simulink model "AGMD"  (R2024b)
settings: Solver=VariableStepAuto  StartTime=0.0  StopTime=10.0  RelTol=1e-3
settings Model: Creator=Jan.Seemann  LastModifiedBy=Jan.Seemann

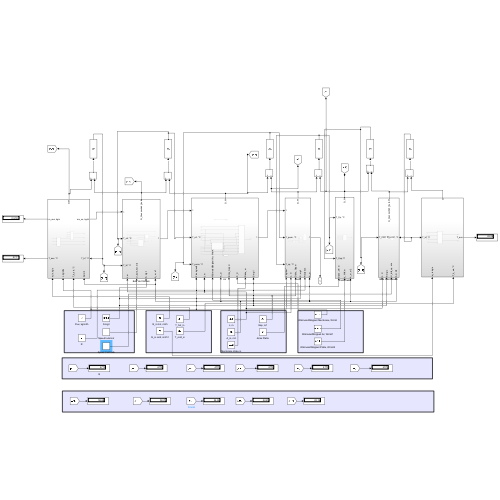
[thumbnail: Simulink's stored preview of the top-level diagram]
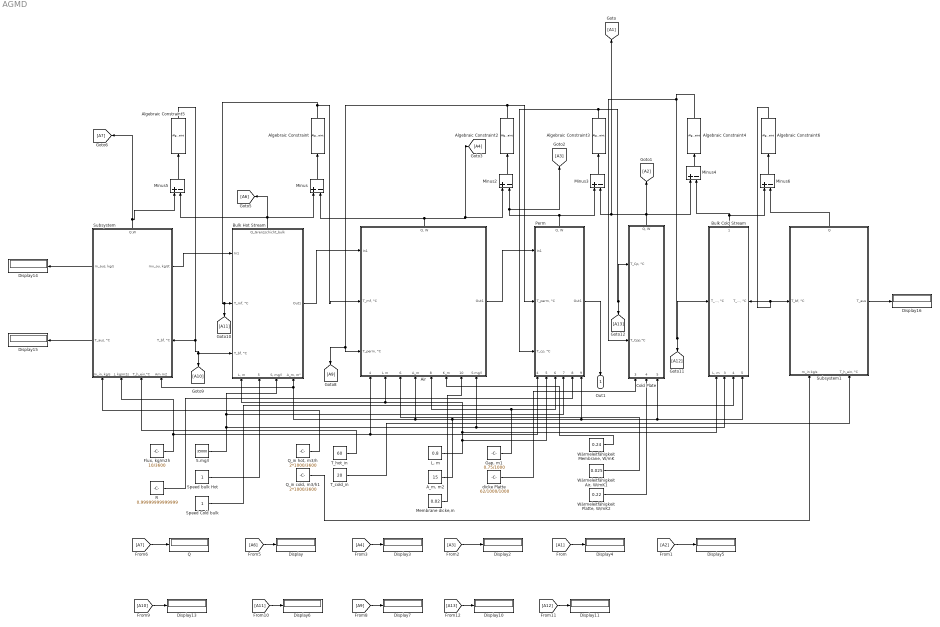
== system AGMD ==
  "A_m, m2" : Constant  Value=15
  Air : Subsystem
      settings: PortSchema="{\"entries\":[{\"content\":{\"sides\":[{\"content\":{\"connectorIds\":[\"In1\",\"In2\",\"In3\"]},\"type\":\"ConnectorPlacement.EquallySpacedRectSide\",\"uuid\":\"bd7e9c2c-f0a2-48a5-8311-5bf6554eac0a\"},{\"content\":{\"connectorIds\":[\"Out1\"],\"side\":\"RIGHT\"},\"type\":\"ConnectorPlacement.EquallySpacedRectSide\",\"uuid\":\"a3684f32-faf2-4467-b21c-0f713c59ca77\"},{\"content\":{\"connectorIds\":[\"Out2\"],\"side\":\"TOP\"},\"type\":\"ConnectorPlacement.EquallySpacedRectSide\",\"uuid\":\"82436852-e058-4df1-b206-5c7722c02e8b\"},{\"content\":{\"connectorIds\":[\"In4\",\"In5\",\"In6\",\"In7\",\"In8\",\"In9\",\"In10\",\"In11\"],\"side\":\"BOTTOM\"},\"type\":\"ConnectorPlacement.EquallySpacedRectSide\",\"uuid\":\"38f1cf92-a27b-45d7-b2e5-179d0ca03cfb\"}]},\"type\":\"ConnectorPlacement.EquallySpacedConnector\",\"uuid\":\"ff56ecae-8895-4e03-a87d-4d8ddd8f3410\"}],\"packageUris\":[\"http://schema.mathworks.com/mf0/Connector/R2020b\"],\"version\":\"1.0\"}"
  Algebraic Constraint{,2..4,6} (5 alike) : AlgebraicConstraint
  Algebraic Constraint5 : AlgebraicConstraint  InitialGuess=1000
  Bulk Cold Stream : Subsystem
      settings: PortSchema="{\"entries\":[{\"content\":{\"sides\":[{\"content\":{\"connectorIds\":[\"In1\"]},\"type\":\"ConnectorPlacement.EquallySpacedRectSide\",\"uuid\":\"e70a48bc-ecb8-4c68-8a9f-c4da01e90966\"},{\"content\":{\"connectorIds\":[\"In6\"],\"side\":\"RIGHT\"},\"type\":\"ConnectorPlacement.EquallySpacedRectSide\",\"uuid\":\"e0687598-31c0-4dfa-b2a4-49cd0c269e12\"},{\"content\":{\"connectorIds\":[\"Out1\"],\"side\":\"TOP\"},\"type\":\"ConnectorPlacement.EquallySpacedRectSide\",\"uuid\":\"e16677ea-1295-45ec-b158-1feb552f65c2\"},{\"content\":{\"connectorIds\":[\"In2\",\"In3\",\"In4\",\"In5\"],\"side\":\"BOTTOM\"},\"type\":\"ConnectorPlacement.EquallySpacedRectSide\",\"uuid\":\"f3e51636-c9ad-451e-9c8a-1e5579e8e767\"}]},\"type\":\"ConnectorPlacement.EquallySpacedConnector\",\"uuid\":\"7ebddd5e-a98a-423c-a868-5fd78b00260d\"}],\"packageUris\":[\"http://schema.mathworks.com/mf0/Connector/R2020b\"],\"version\":\"1.0\"}"
  Bulk Hot Stream : Subsystem
      settings: PortSchema="{\"entries\":[{\"content\":{\"sides\":[{\"content\":{\"connectorIds\":[\"In1\",\"In2\",\"In3\"]},\"type\":\"ConnectorPlacement.EquallySpacedRectSide\",\"uuid\":\"e70a48bc-ecb8-4c68-8a9f-c4da01e90966\"},{\"content\":{\"connectorIds\":[\"Out1\"],\"side\":\"RIGHT\"},\"type\":\"ConnectorPlacement.EquallySpacedRectSide\",\"uuid\":\"e0687598-31c0-4dfa-b2a4-49cd0c269e12\"},{\"content\":{\"connectorIds\":[\"Out2\"],\"side\":\"TOP\"},\"type\":\"ConnectorPlacement.EquallySpacedRectSide\",\"uuid\":\"e16677ea-1295-45ec-b158-1feb552f65c2\"},{\"content\":{\"connectorIds\":[\"In4\",\"In5\",\"In6\",\"In7\"],\"side\":\"BOTTOM\"},\"type\":\"ConnectorPlacement.EquallySpacedRectSide\",\"uuid\":\"ebf15a66-5a6b-483e-aac7-a267298982ca\"}]},\"type\":\"ConnectorPlacement.EquallySpacedConnector\",\"uuid\":\"7ebddd5e-a98a-423c-a868-5fd78b00260d\"}],\"packageUris\":[\"http://schema.mathworks.com/mf0/Connector/R2020b\"],\"version\":\"1.0\"}"
  Cold Plate : Subsystem
      settings: PortSchema="{\"entries\":[{\"content\":{\"sides\":[{\"content\":{\"connectorIds\":[\"In1\",\"In2\"]},\"type\":\"ConnectorPlacement.EquallySpacedRectSide\",\"uuid\":\"9e1ba899-2b74-4207-8077-e6ff28ab6074\"},{\"content\":{\"side\":\"RIGHT\"},\"type\":\"ConnectorPlacement.EquallySpacedRectSide\",\"uuid\":\"ad1c4bce-80e4-42ef-b0be-0137cbf6e500\"},{\"content\":{\"connectorIds\":[\"Out1\"],\"side\":\"TOP\"},\"type\":\"ConnectorPlacement.EquallySpacedRectSide\",\"uuid\":\"d3387212-4e4f-4b7b-acbb-c10cef1fa7fe\"},{\"content\":{\"connectorIds\":[\"In3\",\"In4\",\"In5\"],\"side\":\"BOTTOM\"},\"type\":\"ConnectorPlacement.EquallySpacedRectSide\",\"uuid\":\"8c26ea7c-5b47-4ec8-8354-f3a14176f7be\"}]},\"type\":\"ConnectorPlacement.EquallySpacedConnector\",\"uuid\":\"68209396-1827-4e0e-92d3-38f837a85383\"}],\"packageUris\":[\"http://schema.mathworks.com/mf0/Connector/R2020b\"],\"version\":\"1.0\"}"
  Display{,2..7,10..11,13..16} (13 alike) : Display
  "Flux, kg/m2h" : Constant  Value=10/3600
  "Gap, m1" : Constant  Value=0.75/1000
  "L, m" : Constant  Value=0.8
  Membrane dicke,m : Constant  Value=0.02
  Minus{,2..6} (6 alike) : Sum  Inputs=+-
  Perm : Subsystem
      settings: PortSchema="{\"entries\":[{\"content\":{\"sides\":[{\"content\":{\"connectorIds\":[\"In1\",\"In2\",\"In3\"]},\"type\":\"ConnectorPlacement.EquallySpacedRectSide\",\"uuid\":\"bd7e9c2c-f0a2-48a5-8311-5bf6554eac0a\"},{\"content\":{\"connectorIds\":[\"Out1\"],\"side\":\"RIGHT\"},\"type\":\"ConnectorPlacement.EquallySpacedRectSide\",\"uuid\":\"a3684f32-faf2-4467-b21c-0f713c59ca77\"},{\"content\":{\"connectorIds\":[\"Out2\"],\"side\":\"TOP\"},\"type\":\"ConnectorPlacement.EquallySpacedRectSide\",\"uuid\":\"82436852-e058-4df1-b206-5c7722c02e8b\"},{\"content\":{\"connectorIds\":[\"In4\",\"In5\",\"In6\",\"In7\",\"In8\",\"In9\"],\"side\":\"BOTTOM\"},\"type\":\"ConnectorPlacement.EquallySpacedRectSide\",\"uuid\":\"38f1cf92-a27b-45d7-b2e5-179d0ca03cfb\"}]},\"type\":\"ConnectorPlacement.EquallySpacedConnector\",\"uuid\":\"ff56ecae-8895-4e03-a87d-4d8ddd8f3410\"}],\"packageUris\":[\"http://schema.mathworks.com/mf0/Connector/R2020b\"],\"version\":\"1.0\"}"
  Q : Display
  "Q_in cold, m3/h1" : Constant  Value=2*1000/3600
  "Q_in hot, m3/h" : Constant  Value=2*1000/3600
  R : Constant  Value=0.99999999999999
  S.mg/l : Constant  Value=35000
  Speed Cold bulk : Constant
  Speed bulk Hot : Constant
  Subsystem : Subsystem
      settings: PortSchema="{\"entries\":[{\"content\":{\"sides\":[{\"content\":{\"connectorIds\":[\"Out3\",\"Out4\"]},\"type\":\"ConnectorPlacement.EquallySpacedRectSide\",\"uuid\":\"072a0096-51c0-4f6a-b6c4-abf1e1a1197c\"},{\"content\":{\"connectorIds\":[\"Out1\",\"In5\"],\"side\":\"RIGHT\"},\"type\":\"ConnectorPlacement.EquallySpacedRectSide\",\"uuid\":\"828cba50-d00c-4f62-9248-b6ca73512d1c\"},{\"content\":{\"connectorIds\":[\"Out2\"],\"side\":\"TOP\"},\"type\":\"ConnectorPlacement.EquallySpacedRectSide\",\"uuid\":\"de7aff42-ccc0-4f9f-9cee-8693d471182f\"},{\"content\":{\"connectorIds\":[\"In1\",\"In2\",\"In3\",\"In4\"],\"side\":\"BOTTOM\"},\"type\":\"ConnectorPlacement.EquallySpacedRectSide\",\"uuid\":\"4d4eb3d6-85f7-429f-a39c-e6dd405c8415\"}]},\"type\":\"ConnectorPlacement.EquallySpacedConnector\",\"uuid\":\"4bf11b08-ae68-4af4-a84e-2ff15ce6492f\"}],\"packageUris\":[\"http://schema.mathworks.com/mf0/Connector/R2020b\"],\"version\":\"1.0\"}"
  Subsystem1 : Subsystem
      settings: PortSchema="{\"entries\":[{\"content\":{\"sides\":[{\"content\":{\"connectorIds\":[\"In1\"]},\"type\":\"ConnectorPlacement.EquallySpacedRectSide\",\"uuid\":\"072a0096-51c0-4f6a-b6c4-abf1e1a1197c\"},{\"content\":{\"connectorIds\":[\"Out1\"],\"side\":\"RIGHT\"},\"type\":\"ConnectorPlacement.EquallySpacedRectSide\",\"uuid\":\"828cba50-d00c-4f62-9248-b6ca73512d1c\"},{\"content\":{\"connectorIds\":[\"Out2\"],\"side\":\"TOP\"},\"type\":\"ConnectorPlacement.EquallySpacedRectSide\",\"uuid\":\"de7aff42-ccc0-4f9f-9cee-8693d471182f\"},{\"content\":{\"connectorIds\":[\"In2\",\"In3\"],\"side\":\"BOTTOM\"},\"type\":\"ConnectorPlacement.EquallySpacedRectSide\",\"uuid\":\"4d4eb3d6-85f7-429f-a39c-e6dd405c8415\"}]},\"type\":\"ConnectorPlacement.EquallySpacedConnector\",\"uuid\":\"4bf11b08-ae68-4af4-a84e-2ff15ce6492f\"}],\"packageUris\":[\"http://schema.mathworks.com/mf0/Connector/R2020b\"],\"version\":\"1.0\"}"
  T_cold_in : Constant  Value=20
  T_hot_in : Constant  Value=60
  "Wärmeleitfähigkeit Air, W/mK1" : Constant  Value=0.025
  "Wärmeleitfähigkeit Membrane, W/mK" : Constant  Value=0.24
  "Wärmeleitfähigkeit Platte, W/mK2" : Constant  Value=0.22
  dicke Platte : Constant  Value=62/1000/1000
  Out1 : Outport
  wires:
  Bulk Hot Stream/2(Q_Grenzschicht_bulk) -> [A6], Minus/1, Minus5/2
  Minus/1 -> Algebraic Constraint/1
  Algebraic Constraint/1 -> Air/2("T_mf, °C"), [A11], Bulk Hot Stream/2("T_mf, °C")
  Air/2("Q, W") -> Minus/2, Minus2/1, [A4]
  Minus2/1 -> Algebraic Constraint2/1
  Perm/2("Q, W") -> Minus3/1, [A3], Minus2/2
  Algebraic Constraint2/1 -> Perm/2("T_perm, °C"), Air/3("T_perm, °C"), [A9]
  Minus3/1 -> Algebraic Constraint3/1
  Cold Plate/1("Q, W") -> Minus4/1, [A2], Minus3/2, [A1]
  Algebraic Constraint3/1 -> [A13], Cold Plate/1("T_Cp, °C"), Perm/3("T_cp, °C")
  Minus4/1 -> Algebraic Constraint4/1
  Bulk Cold Stream/1("Q_Grenzschicht_bulk, W") -> Minus6/1, Minus4/2
  Algebraic Constraint4/1 -> [A12], Bulk Cold Stream/1("T_CPP, °C"), Cold Plate/2(T_Cpp,°C)
  Minus5/1 -> Algebraic Constraint5/1
  Subsystem/2(Q,W) -> [A7], Minus5/1
  Algebraic Constraint5/1 -> [A10], Bulk Hot Stream/3("T_bf, °C"), Subsystem/5("T_bf, °C")
  Subsystem/3("m_aus, kg/s") -> Display14/1
  Subsystem/4("T_aus, °C") -> Display15/1
  Algebraic Constraint6/1 -> Bulk Cold Stream/6("T_bf-CP, °C"), Subsystem1/1("T_bf, °C")
  Minus6/1 -> Algebraic Constraint6/1
  Subsystem1/2(Q) -> Minus6/2
  Subsystem1/1(T_aus) -> Display16/1
  [A1] -> Display4/1
  [A2] -> Display5/1
  [A3] -> Display2/1
  [A4] -> Display3/1
  [A6] -> Display/1
  [A7] -> Q/1
  [A9] -> Display7/1
  [A10] -> Display13/1
  [A11] -> Display6/1
  [A12] -> Display11/1
  [A13] -> Display10/1
  Subsystem/1("mx_ou, kg/st") -> Bulk Hot Stream/1(In1)
  Bulk Hot Stream/1(Out1) -> Air/1(In1)
  Air/1(Out1) -> Perm/1(In1)
  Perm/1(Out1) -> Out1/1
  "Q_in hot, m3/h"/1 -> Subsystem/1("m_in, kg/s")
  S.mg/l/1 -> Air/11(S mg/l), Bulk Cold Stream/3(S mg/L), Perm/7("S, mg/l"), Bulk Hot Stream/6("S, mg/l")
  "A_m, m2"/1 -> Subsystem/4(Am m2), Bulk Hot Stream/7("A_m, m\""), Air/7(A_m), Bulk Cold Stream/5("Am, m2"), Cold Plate/5("A_m, m2"), Perm/9(A_m)
  "Gap, m1"/1 -> Perm/6(Dicke_Gap m), Air/8(dicke_Gap m)
  dicke Platte/1 -> Cold Plate/3("Dicke_CP, m")
  Membrane dicke,m/1 -> Air/10(Dicke_m)
  "L, m"/1 -> Bulk Cold Stream/2("L, m"), Bulk Hot Stream/4("L, m"), Air/5(L m), Perm/5("L, m")
  T_hot_in/1 -> Subsystem/3(T_h_ein,°C)
  Speed bulk Hot/1 -> Bulk Hot Stream/5("U_bulk_hot, m/s")
  Speed Cold bulk/1 -> Bulk Cold Stream/4("U_bilk_cp, m/s")
  R/1 -> Perm/8(Recjetion)
  "Flux, kg/m2h"/1 -> Perm/4("J kg/hm\""), Air/4(Flux kg/sm2), Subsystem/2("J, kg/m2s")
  "Wärmeleitfähigkeit Platte, W/mK2"/1 -> Cold Plate/4(k_W/Km)
  "Wärmeleitfähigkeit Air, W/mK1"/1 -> Air/6("Wärmeleitfähigkeit Air, W/mK")
  "Wärmeleitfähigkeit Membrane, W/mK"/1 -> Air/9(K_m)
  "Q_in cold, m3/h1"/1 -> Subsystem1/2(m_in kg/s)
  T_cold_in/1 -> Subsystem1/3("T_h_ein, °C")

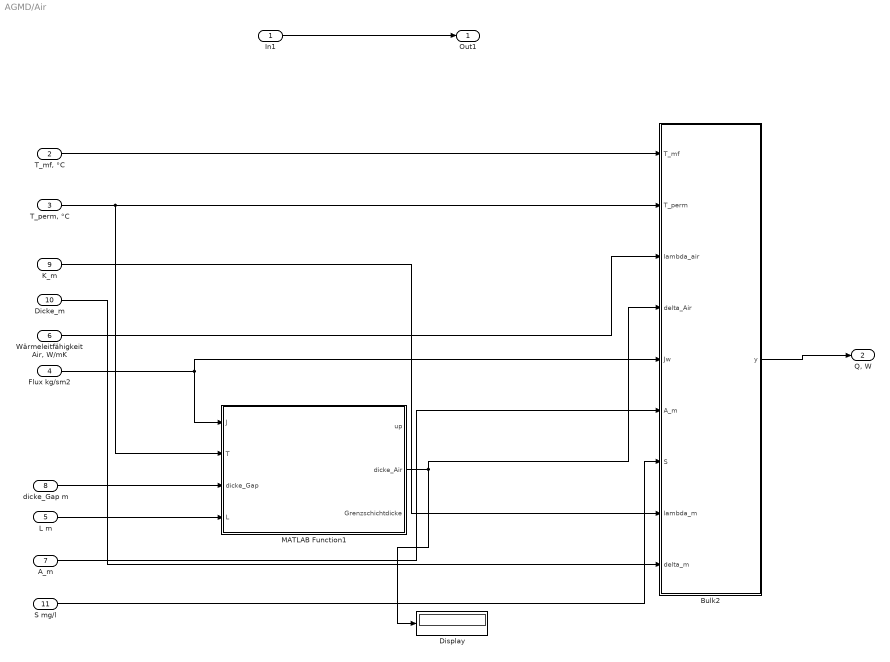
== system AGMD/Air ==
  In1 : Inport
  "T_mf, °C" : Inport  Port=2
  "T_perm, °C" : Inport  Port=3
  Flux kg/sm2 : Inport  Port=4
  L m : Inport  Port=5
  "Wärmeleitfähigkeit Air, W/mK" : Inport  Port=6
  A_m : Inport  Port=7
  dicke_Gap m : Inport  Port=8
  K_m : Inport  Port=9
  Dicke_m : Inport  Port=10
  S mg/l : Inport  Port=11
  Bulk2 : MATLAB Function  TreatAsAtomicUnit=on
  Display : Display
  MATLAB Function1 : MATLAB Function  TreatAsAtomicUnit=on
  Out1 : Outport
  "Q, W" : Outport  Port=2
  wires:
  In1/1 -> Out1/1
  Flux kg/sm2/1 -> Bulk2/5(Jw), MATLAB Function1/1(J)
  "T_perm, °C"/1 -> MATLAB Function1/2(T), Bulk2/2(T_perm)
  "Wärmeleitfähigkeit Air, W/mK"/1 -> Bulk2/3(lambda_air)
  "T_mf, °C"/1 -> Bulk2/1(T_mf)
  Bulk2/1(y) -> "Q, W"/1
  A_m/1 -> Bulk2/6(A_m)
  L m/1 -> MATLAB Function1/4(L)
  dicke_Gap m/1 -> MATLAB Function1/3(dicke_Gap)
  K_m/1 -> Bulk2/8(lambda_m)
  Dicke_m/1 -> Bulk2/9(delta_m)
  MATLAB Function1/2(dicke_Air) -> Display/1, Bulk2/4(delta_Air)
  S mg/l/1 -> Bulk2/7(S)

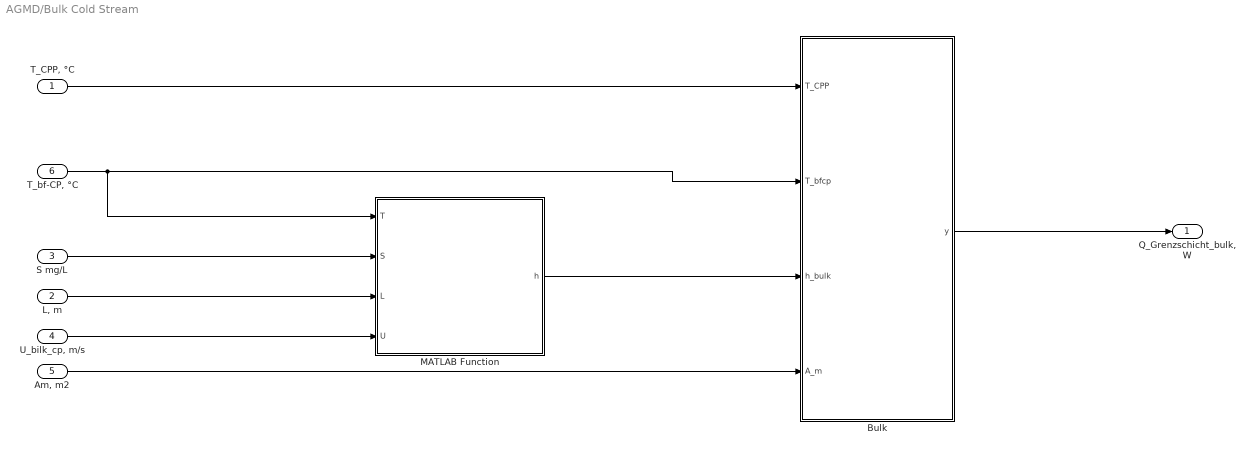
== system AGMD/Bulk Cold Stream ==
  "T_CPP, °C" : Inport
  "L, m" : Inport  Port=2
  S mg/L : Inport  Port=3
  "U_bilk_cp, m/s" : Inport  Port=4
  "Am, m2" : Inport  Port=5
  "T_bf-CP, °C" : Inport  Port=6
  Bulk : MATLAB Function  TreatAsAtomicUnit=on
  MATLAB Function : MATLAB Function  TreatAsAtomicUnit=on
  "Q_Grenzschicht_bulk, W" : Outport
  wires:
  MATLAB Function/1(h) -> Bulk/3(h_bulk)
  "T_CPP, °C"/1 -> Bulk/1(T_CPP)
  "T_bf-CP, °C"/1 -> MATLAB Function/1(T), Bulk/2(T_bfcp)
  Bulk/1(y) -> "Q_Grenzschicht_bulk, W"/1
  S mg/L/1 -> MATLAB Function/2(S)
  "L, m"/1 -> MATLAB Function/3(L)
  "U_bilk_cp, m/s"/1 -> MATLAB Function/4(U)
  "Am, m2"/1 -> Bulk/4(A_m)

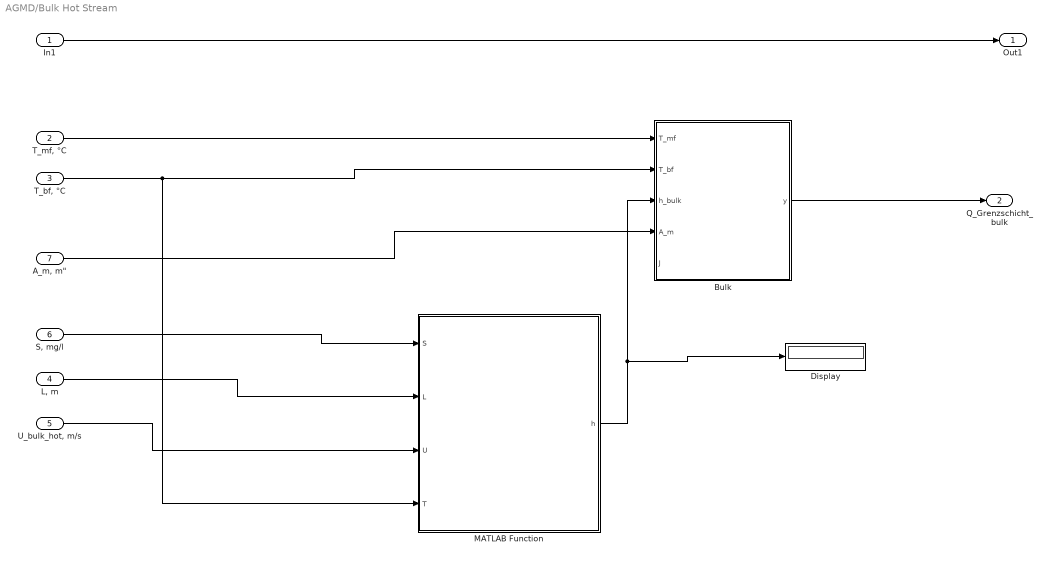
== system AGMD/Bulk Hot Stream ==
  In1 : Inport
  "T_mf, °C" : Inport  Port=2
  "T_bf, °C" : Inport  Port=3
  "L, m" : Inport  Port=4
  "U_bulk_hot, m/s" : Inport  Port=5
  "S, mg/l" : Inport  Port=6
  "A_m, m\"" : Inport  Port=7
  Bulk : MATLAB Function  TreatAsAtomicUnit=on
  Display : Display
  MATLAB Function : MATLAB Function  TreatAsAtomicUnit=on
  Out1 : Outport
  Q_Grenzschicht_bulk : Outport  Port=2
  wires:
  In1/1 -> Out1/1
  MATLAB Function/1(h) -> Display/1, Bulk/3(h_bulk)
  "T_mf, °C"/1 -> Bulk/1(T_mf)
  "T_bf, °C"/1 -> MATLAB Function/4(T), Bulk/2(T_bf)
  Bulk/1(y) -> Q_Grenzschicht_bulk/1
  "S, mg/l"/1 -> MATLAB Function/1(S)
  "L, m"/1 -> MATLAB Function/2(L)
  "U_bulk_hot, m/s"/1 -> MATLAB Function/3(U)
  "A_m, m\""/1 -> Bulk/4(A_m)

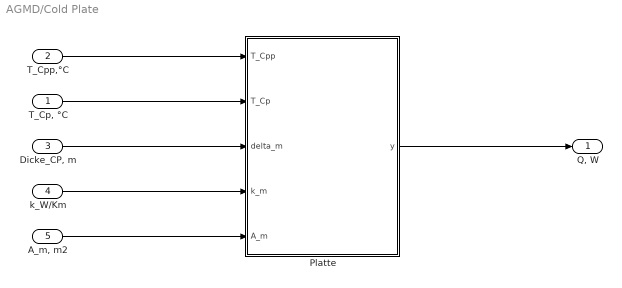
== system AGMD/Cold Plate ==
  "T_Cp, °C" : Inport
  T_Cpp,°C : Inport  Port=2
  "Dicke_CP, m" : Inport  Port=3
  k_W/Km : Inport  Port=4
  "A_m, m2" : Inport  Port=5
  Platte : MATLAB Function  TreatAsAtomicUnit=on
  "Q, W" : Outport
  wires:
  T_Cpp,°C/1 -> Platte/1(T_Cpp)
  "T_Cp, °C"/1 -> Platte/2(T_Cp)
  "Dicke_CP, m"/1 -> Platte/3(delta_m)
  Platte/1(y) -> "Q, W"/1
  k_W/Km/1 -> Platte/4(k_m)
  "A_m, m2"/1 -> Platte/5(A_m)

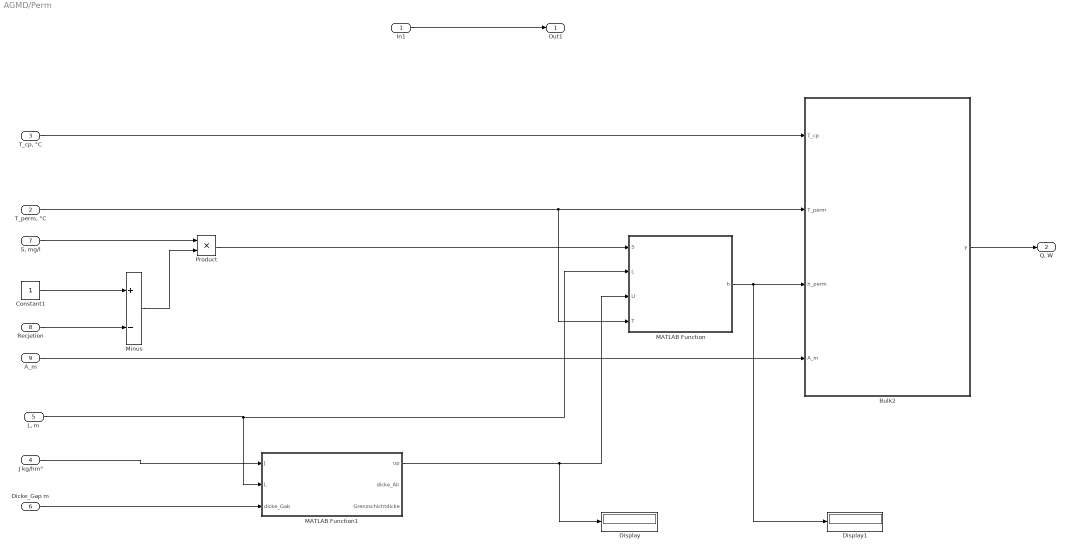
== system AGMD/Perm ==
  In1 : Inport
  "T_perm, °C" : Inport  Port=2
  "T_cp, °C" : Inport  Port=3
  "J kg/hm\"" : Inport  Port=4
  "L, m" : Inport  Port=5
  Dicke_Gap m : Inport  Port=6
  "S, mg/l" : Inport  Port=7
  Recjetion : Inport  Port=8
  A_m : Inport  Port=9
  Bulk2 : MATLAB Function  TreatAsAtomicUnit=on
  Constant1 : Constant
  Display : Display
  Display1 : Display
  MATLAB Function : MATLAB Function  TreatAsAtomicUnit=on
  MATLAB Function1 : MATLAB Function  TreatAsAtomicUnit=on
  Minus : Sum  Inputs=+-
  Product : Product
  Out1 : Outport
  "Q, W" : Outport  Port=2
  wires:
  In1/1 -> Out1/1
  "T_cp, °C"/1 -> Bulk2/1(T_cp)
  Bulk2/1(y) -> "Q, W"/1
  "T_perm, °C"/1 -> MATLAB Function/4(T), Bulk2/2(T_perm)
  MATLAB Function1/1(up) -> Display/1, MATLAB Function/3(U)
  "L, m"/1 -> MATLAB Function1/2(L), MATLAB Function/2(L)
  Product/1 -> MATLAB Function/1(S)
  Constant1/1 -> Minus/1
  Recjetion/1 -> Minus/2
  Minus/1 -> Product/2
  "S, mg/l"/1 -> Product/1
  MATLAB Function/1(h) -> Display1/1, Bulk2/3(h_perm)
  Dicke_Gap m/1 -> MATLAB Function1/3(dicke_Gab)
  A_m/1 -> Bulk2/4(A_m)
  "J kg/hm\""/1 -> MATLAB Function1/1(J)

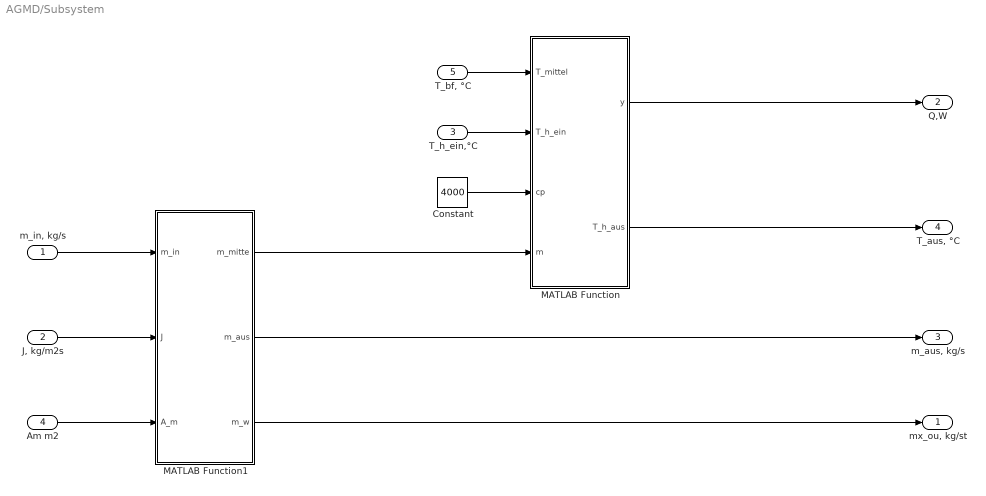
== system AGMD/Subsystem ==
  "m_in, kg/s" : Inport
  "J, kg/m2s" : Inport  Port=2
  T_h_ein,°C : Inport  Port=3
  Am m2 : Inport  Port=4
  "T_bf, °C" : Inport  Port=5
  Constant : Constant  Value=4000
  MATLAB Function : MATLAB Function  TreatAsAtomicUnit=on
  MATLAB Function1 : MATLAB Function  TreatAsAtomicUnit=on
  "mx_ou, kg/st" : Outport
  Q,W : Outport  Port=2
  "m_aus, kg/s" : Outport  Port=3
  "T_aus, °C" : Outport  Port=4
  wires:
  MATLAB Function1/1(m_mitte) -> MATLAB Function/4(m)
  MATLAB Function1/2(m_aus) -> "m_aus, kg/s"/1
  "J, kg/m2s"/1 -> MATLAB Function1/2(J)
  Constant/1 -> MATLAB Function/3(cp)
  T_h_ein,°C/1 -> MATLAB Function/2(T_h_ein)
  "T_bf, °C"/1 -> MATLAB Function/1(T_mittel)
  MATLAB Function/1(y) -> Q,W/1
  MATLAB Function/2(T_h_aus) -> "T_aus, °C"/1
  Am m2/1 -> MATLAB Function1/3(A_m)
  MATLAB Function1/3(m_w) -> "mx_ou, kg/st"/1
  "m_in, kg/s"/1 -> MATLAB Function1/1(m_in)

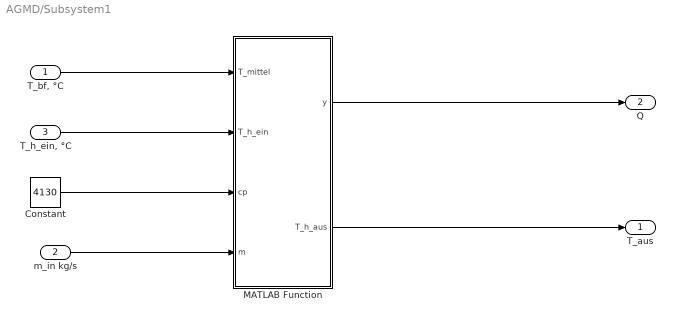
== system AGMD/Subsystem1 ==
  "T_bf, °C" : Inport
  m_in kg/s : Inport  Port=2
  "T_h_ein, °C" : Inport  Port=3
  Constant : Constant  Value=4130
  MATLAB Function : MATLAB Function  TreatAsAtomicUnit=on
  T_aus : Outport
  Q : Outport  Port=2
  wires:
  m_in kg/s/1 -> MATLAB Function/4(m)
  Constant/1 -> MATLAB Function/3(cp)
  "T_h_ein, °C"/1 -> MATLAB Function/2(T_h_ein)
  "T_bf, °C"/1 -> MATLAB Function/1(T_mittel)
  MATLAB Function/1(y) -> Q/1
  MATLAB Function/2(T_h_aus) -> T_aus/1

== matlab function AGMD/Perm/Bulk2 ==
  data: T_cp input; T_perm input; y output; h_perm input; A_m input
function y = fcn(T_cp,T_perm, h_perm,A_m)

y = A_m * h_perm * (T_perm -T_cp ) ;

== matlab function AGMD/Air/Bulk2 ==
  data: T_mf input; T_perm input; y output; lambda_air input; delta_Air input; Jw input; A_m input; S input; lambda_m input; delta_m input
function y = fcn(T_mf,T_perm, lambda_air,delta_Air,Jw,A_m,S , lambda_m, delta_m)

T_mitte = (T_mf + T_perm)/2 + 273.15;
% Cp = 4000;
Hw = (1.75535 * T_mitte + 2024.3);
% hy = lambda_air/delta_Air;
% h = ( Jw * Cp ) / ( 1 - exp (-Jw*Cp /hy));

T = (T_mf + T_perm)/2;

    S_kgkg = S / 1000 /1000;

    % Korrelation für reines Wasser (in J/kg)
    h_fg_w = (2.501e6 - 2.361e3 * T);

    % Korrekturfaktor für Salzgehalt
    delta_h = (0.0158 * S_kgkg + 0.00012 * S_kgkg.^2) * 1e6;

    % Verdampfungsenthalpie von Meerwasser
    h_fg_sw = h_fg_w - delta_h;


    h = (delta_Air/lambda_air + delta_m / lambda_m)^(-1);

y = A_m * (T_mf - T_perm)* h + Jw *A_m *Hw ;

== matlab function AGMD/Subsystem/MATLAB Function1 ==
  data: m_in input; m_mitte output; J input; m_aus output; A_m input; m_w output
function [m_mitte,m_aus,m_w] = fcn(m_in,J,A_m)

m_aus = m_in - J *A_m;        % Massenbilanz zur ermittlung der Masse aus (Brine) [kg/s]
m_mitte = (m_in + m_aus)/2 ;  % mittlere Masse [kg/s]
m_w = J *A_m;                 % Masse Perm [kg/s]

== matlab function AGMD/Cold Plate/Platte ==
  data: T_Cpp input; y output; T_Cp input; delta_m input; k_m input; A_m input
function y = fcn(T_Cpp, T_Cp , delta_m,k_m,A_m)
% Membrangeometrie



y = A_m*  k_m/delta_m *(T_Cp - T_Cpp);

== matlab function AGMD/Subsystem1/MATLAB Function ==
  data: T_mittel input; y output; T_h_ein input; cp input; m input; T_h_aus output
function [y ,T_h_aus] = fcn(T_mittel, T_h_ein,cp,m)



T_h_aus = T_mittel*2 - T_h_ein;


y = cp * m * (T_h_aus - T_h_ein);

== matlab function AGMD/Bulk Hot Stream/Bulk ==
  data: T_mf input; y output; T_bf input; h_bulk input; A_m input; J input
function y = fcn(T_mf, T_bf, h_bulk,A_m, J)
T_mitte = (T_mf + T_bf)/2 + 273.15;

Hw = (1.75535 * T_mitte + 2024.3)*1000;
y = A_m * h_bulk * (T_bf - T_mf) + J * A_m * Hw;

== matlab function AGMD/Bulk Cold Stream/Bulk ==
  data: T_CPP input; y output; T_bfcp input; h_bulk input; A_m input
function y = fcn(T_CPP , T_bfcp, h_bulk,A_m)
% Membrangeometrie
A_m = 1.6;              % Membranfläche [m^2]
delta_m = 0.4e-3;       % Membrandicke [m]
delta_a = 2e-3;         % Air-gap Dicke [m]
delta_cp = 1.5e-3;      % Kühlplattenstärke [m]

% Wärmeleitfähigkeiten
k_m = 0.2;              % Membran [W/mK]
k_a = 0.03;             % Luft [W/mK]
k_cp = 60;              % Kühlplatte [W/mK]



y = A_m * h_bulk * (T_CPP-T_bfcp) ;

== matlab function AGMD/Bulk Hot Stream/MATLAB Function ==
  data: S input; L input; U input; T input; h output
function h = h_plate_meerwasser( S, L, U, T)
% Berechnet den Wärmeübergangskoeffizienten h [W/m^2K]
% für Meerwasser an einer ebenen Platte bei paralleler Umströmung
%
% Eingabeparameter:
% T  - Temperatur in °C
% S  - Salzgehalt in g/kg
% L  - charakteristische Länge der Platte in m
% U  - Strömungsgeschwindigkeit in m/s
%
% Ausgabe:
% h  - Wärmeübergangskoeffizient in W/m²K
if T > 120
    T = 60;
end
S = S /1000; % von mg/l in g/kg

% --- Schritt 1: Materialeigenschaften für Meerwasser ---
% Näherungsweise: empirische Gleichungen aus Sharqawy et al. (Desalination, 2010)

rho = 1000 -0.07*S + 0.2*T;         % Dichte [kg/m³]
mu = (1e-3)*(1 + 0.02*S/35 - 0.033*T/25);  % Viskosität [Pa·s] vereinfacht
cp = 4180 - 10*S;                    % Wärmekapazität [J/kg·K]
k = 0.6 - 0.001*T;                   % Wärmeleitfähigkeit [W/m·K]

% --- Schritt 2: Kenngrößen ---
nu = mu / rho;                      % Kinematische Viskosität [m²/s]
alpha = k / (rho * cp);            % Temperaturleitfähigkeit [m²/s]
Pr = nu / alpha;                   % Prandtl-Zahl
Re = U * L / nu;                   % Reynolds-Zahl

% --- Schritt 3: Nusselt-Zahl berechnen ---
if Re < 5e5
    Nu = 0.664 * Re^0.5 * Pr^(1/3);    % laminare Strömung (mittlerer Nu)
else
    Nu = 0.037 * Re^0.8 * Pr^(1/3);    % turbulente Strömung
end

% --- Schritt 4: Wärmeübergangskoeffizient ---
h = Nu * k / L;                      % [W/m²K]

end

== matlab function AGMD/Bulk Cold Stream/MATLAB Function ==
  data: T input; S input; L input; U input; h output
function h = h_plate_meerwasser(T, S, L, U)
% Berechnet den Wärmeübergangskoeffizienten h [W/m^2K]
% für Meerwasser an einer ebenen Platte bei paralleler Umströmung
%
% Eingabeparameter:
% T  - Temperatur in °C
% S  - Salzgehalt in g/kg
% L  - charakteristische Länge der Platte in m
% U  - Strömungsgeschwindigkeit in m/s
%
% Ausgabe:
% h  - Wärmeübergangskoeffizient in W/m²K

S = S/1000; % mg/l in g/kg


% --- Schritt 1: Materialeigenschaften für Meerwasser ---
% Näherungsweise: empirische Gleichungen aus Sharqawy et al. (Desalination, 2010)

rho = 1000 - 0.07*S + 0.2*T;         % Dichte [kg/m³]
mu = (1e-3)*(1 + 0.02*S/35 - 0.033*T/25);  % Viskosität [Pa·s] vereinfacht
cp = 4180 - 10*S;                    % Wärmekapazität [J/kg·K]
k = 0.6 - 0.001*T;                   % Wärmeleitfähigkeit [W/m·K]

% --- Schritt 2: Kenngrößen ---
nu = mu / rho;                      % Kinematische Viskosität [m²/s]
alpha = k / (rho * cp);            % Temperaturleitfähigkeit [m²/s]
Pr = nu / alpha;                   % Prandtl-Zahl
Re = U * L / nu;                   % Reynolds-Zahl

% --- Schritt 3: Nusselt-Zahl berechnen ---
if Re < 5e5
    Nu = 0.664 * Re^0.5 * Pr^(1/3);    % laminare Strömung (mittlerer Nu)
else
    Nu = 0.037 * Re^0.8 * Pr^(1/3);    % turbulente Strömung
end

% --- Schritt 4: Wärmeübergangskoeffizient ---
h = Nu * k / L;                      % [W/m²K]

end

== matlab function AGMD/Air/MATLAB Function1 ==
  data: J input; up output; T input; dicke_Air output; Grenzschichtdicke output; dicke_Gap input; L input
function [up, dicke_Air,Grenzschichtdicke]= fcn(J,T,dicke_Gap,L)

%dicke_Gab = 0.05;
%L  = 0.1      ; % m2
nu = 0.467e-3 ; % Pas
Dichte = 983  ; % kg/m3
%J = 12; 
g = 9.81 ; %m/s

Grenzschichtdicke = (3*J*nu*L/(Dichte*Dichte*g))^(1/3);
up = 1/3 * Dichte * g * Grenzschichtdicke^2 / nu;

dicke_Air = dicke_Gap -Grenzschichtdicke;

== matlab function AGMD/Perm/MATLAB Function ==
  data: S input; L input; U input; T input; h output
function h = h_plate_meerwasser( S, L, U, T)
% Berechnet den Wärmeübergangskoeffizienten h [W/m^2K]
% für Meerwasser an einer ebenen Platte bei paralleler Umströmung
%
% Eingabeparameter:
% T  - Temperatur in °C
% S  - Salzgehalt in g/kg
% L  - charakteristische Länge der Platte in m
% U  - Strömungsgeschwindigkeit in m/s
%
% Ausgabe:
% h  - Wärmeübergangskoeffizient in W/m²K

% --- Schritt 1: Materialeigenschaften für Meerwasser ---
% Näherungsweise: empirische Gleichungen aus Sharqawy et al. (Desalination, 2010)
S = S/1000; % umrechnung mg/l in g/kg

rho = 1000 - 0.07*S + 0.2*T;         % Dichte [kg/m³]
mu = (1e-3)*(1 + 0.02*S/35 - 0.033*T/25);  % Viskosität [Pa·s] vereinfacht
cp = 4180 - 10*S;                    % Wärmekapazität [J/kg·K]
k = 0.6 - 0.001*T;                   % Wärmeleitfähigkeit [W/m·K]

% --- Schritt 2: Kenngrößen ---
nu = mu / rho;                      % Kinematische Viskosität [m²/s]
alpha = k / (rho * cp);            % Temperaturleitfähigkeit [m²/s]
Pr = nu / alpha;                   % Prandtl-Zahl
Re = U * L / nu;                   % Reynolds-Zahl

% --- Schritt 3: Nusselt-Zahl berechnen ---
if Re < 5e5
    Nu = 0.664 * Re^0.5 * Pr^(1/3);    % laminare Strömung (mittlerer Nu)
else
    Nu = 0.037 * Re^0.8 * Pr^(1/3);    % turbulente Strömung
end

% --- Schritt 4: Wärmeübergangskoeffizient ---
h = Nu * k / L;                      % [W/m²K]

end

== matlab function AGMD/Perm/MATLAB Function1 ==
  data: J input; up output; dicke_Air output; Grenzschichtdicke output; L input; dicke_Gab input
function [up, dicke_Air,Grenzschichtdicke]= fcn(J,L, dicke_Gab)



nu = 0.467e-3 ; % Pas
Dichte = 983  ; % kg/m3
%J = 12; 
g = 9.81 ; %m/s2

Grenzschichtdicke = (3*J*nu*L/(Dichte*Dichte*g))^(1/3);
up = 1/3 * Dichte * g * Grenzschichtdicke^2 / nu; 

dicke_Air = dicke_Gab -Grenzschichtdicke;

== matlab function AGMD/Subsystem/MATLAB Function ==
  data: T_mittel input; y output; T_h_ein input; cp input; m input; T_h_aus output
function [y ,T_h_aus] = fcn(T_mittel, T_h_ein,cp,m)



T_h_aus = T_mittel*2 - T_h_ein;


y = cp * m * (T_h_ein - T_h_aus);
